simulink model "PLL3_XNOR"  (R2019b)
settings: Solver=ode23  StartTime=0.0  StopTime=tstop  RelTol=1e-5
values from neighbouring files (symbols this model uses):
  dw = 0.1    [LAB2_script.m]
  Kvco = 1    [LAB2_script.m]
  tau = 0.5    [LAB2_script.m]
  w0 = 1e3    (= 1000)    [LAB2_script.m]
  wfr = w0    (= 1000)    [LAB2_script.m]
settings Model: Creator=franc  LastModifiedBy=franc

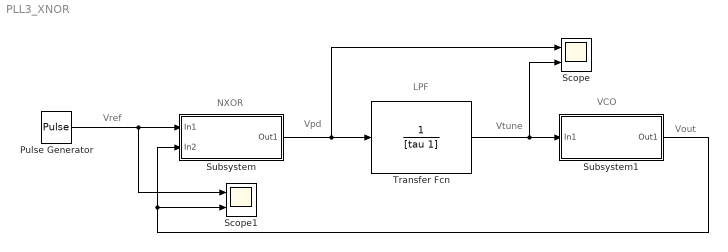
== system PLL3_XNOR ==
  note: Vout
  note: Vtune
  note: Vpd
  note: Vref
  note: VCO
  note: LPF
  note: NXOR
  Pulse Generator : DiscretePulseGenerator  PulseType=Time based  Period=2*pi/(w0+dw)  PulseWidth=50
  Scope : Scope  NumInputPorts=2
  Scope1 : Scope  NumInputPorts=2
  Subsystem : Subsystem
  Subsystem1 : Subsystem
  Transfer Fcn : TransferFcn  Denominator=[tau 1]
  wires:
  Pulse Generator/1 -> Scope1/1, Subsystem/1(In1)
  Subsystem/1(Out1) -> Scope/1, Transfer Fcn/1
  Subsystem1/1(Out1) -> Scope1/2, Subsystem/2(In2)
  Transfer Fcn/1 -> Scope/2, Subsystem1/1(In1)

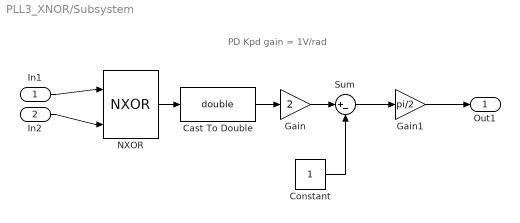
== system PLL3_XNOR/Subsystem ==
  note: PD Kpd gain = 1V/rad
  In1 : Inport
  In2 : Inport  Port=2
  Cast To Double : DataTypeConversion  OutDataTypeStr=double
  Constant : Constant
  Gain : Gain  Gain=2
  Gain1 : Gain  Gain=pi/2
  NXOR : Logic  Operator=NXOR  IconShape=distinctive  AllPortsSameDT=off  OutDataTypeStr=boolean
  Sum : Sum  Inputs=|+-
  Out1 : Outport
  wires:
  In1/1 -> NXOR/1
  In2/1 -> NXOR/2
  NXOR/1 -> Cast To Double/1
  Cast To Double/1 -> Gain/1
  Gain/1 -> Sum/1
  Constant/1 -> Sum/2
  Sum/1 -> Gain1/1
  Gain1/1 -> Out1/1

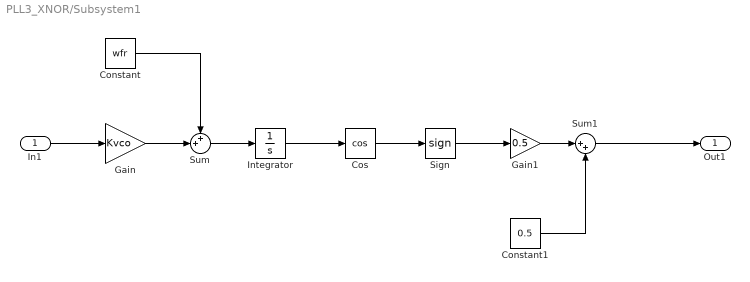
== system PLL3_XNOR/Subsystem1 ==
  In1 : Inport
  Constant : Constant  Value=wfr
  Constant1 : Constant  Value=0.5
  Cos : Trigonometry  Operator=cos
  Gain : Gain  Gain=Kvco
  Gain1 : Gain  Gain=0.5
  Integrator : Integrator
  Sign : Signum
  Sum : Sum  Inputs=++|
  Sum1 : Sum  Inputs=|++
  Out1 : Outport
  wires:
  In1/1 -> Gain/1
  Gain/1 -> Sum/2
  Constant/1 -> Sum/1
  Sum/1 -> Integrator/1
  Integrator/1 -> Cos/1
  Gain1/1 -> Sum1/1
  Constant1/1 -> Sum1/2
  Sum1/1 -> Out1/1
  Cos/1 -> Sign/1
  Sign/1 -> Gain1/1
